simulink model "untitled"  (R2016b)
settings: Solver=VariableStepAuto  StartTime=0.0  StopTime=10.0  RelTol=1e-3
undefined symbols (not defined in the file or in its folder): h
libraries: xbsIndex_r4 x133
settings Model: Creator=rm101  LastModifiedBy=rm101

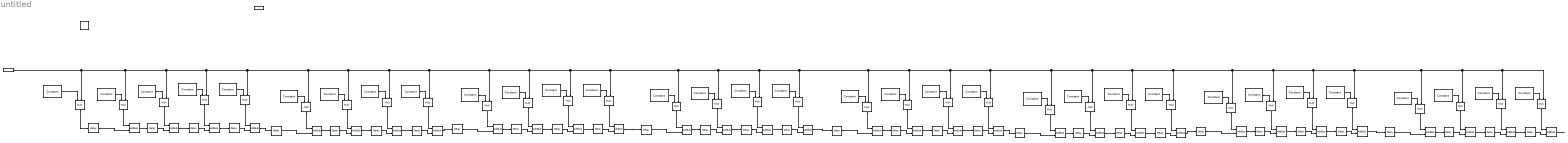
== system untitled ==
  " System Generator" : xbsIndex_r4/ System Generator  Tag=genX  xilinxfamily=Kintex7  part=xc7k325t  speed=-3  package=fbg676  synthesis_tool=Vivado  clock_wrapper=Clock Enables  directory=./netlist  proj_type=Vivado  Synth_file=Vivado Synthesis Defaults  Impl_file=Vivado Implementation Defaults  testbench=off  simulink_period=1  sysclk_period=10  dcm_input_clock_period=10  incr_netlist=off  trim_vbits=Everywhere in SubSystem  dbl_ovrd=According to Block Masks  core_generation=According to Block Masks  run_coregen=off  deprecated_control=off  eval_field=0  block_type=sysgen
  AddSub{,1..31} (32 alike) : xbsIndex_r4/AddSub  mode=Addition  use_carryin=off  use_carryout=off  en=off  latency=add1  precision=Full  arith_type=Unsigned  n_bits=16  bin_pt=14  quantization=Truncate  overflow=Wrap  use_behavioral_HDL=off  hw_selection=Fabric  pipelined=off  dbl_ovrd=off  block_type=addsub
  Constant : xbsIndex_r4/Constant  const=h(16,33)  gui_display_data_type=Fixed-point  arith_type=Signed (2's comp)  n_bits=w  bin_pt=d  preci_type=Single  exp_width=8  frac_width=24  explicit_period=off  period=1  equ=P=C  opselect=C  inp2=PCIN>>17  opr=+  inp1=P  carry=CIN  dbl_ovrd=off  block_type=constant
  Constant{1,5,9,13,17,21,28,32} (8 alike) : xbsIndex_r4/Constant  const=h(16,32)  gui_display_data_type=Fixed-point  arith_type=Signed (2's comp)  n_bits=w  bin_pt=d  preci_type=Single  exp_width=8  frac_width=24  explicit_period=off  period=1  equ=P=C  opselect=C  inp2=PCIN>>17  opr=+  inp1=P  carry=CIN  dbl_ovrd=off  block_type=constant
  Constant{2,6,10,14,18,22,25,29} (8 alike) : xbsIndex_r4/Constant  const=h(16,31)  gui_display_data_type=Fixed-point  arith_type=Signed (2's comp)  n_bits=w  bin_pt=d  preci_type=Single  exp_width=8  frac_width=24  explicit_period=off  period=1  equ=P=C  opselect=C  inp2=PCIN>>17  opr=+  inp1=P  carry=CIN  dbl_ovrd=off  block_type=constant
  Constant{3,7,11,15,19,23,26,30} (8 alike) : xbsIndex_r4/Constant  const=h(16,30)  gui_display_data_type=Fixed-point  arith_type=Signed (2's comp)  n_bits=w  bin_pt=d  preci_type=Single  exp_width=8  frac_width=24  explicit_period=off  period=1  equ=P=C  opselect=C  inp2=PCIN>>17  opr=+  inp1=P  carry=CIN  dbl_ovrd=off  block_type=constant
  Constant{4,8,12,16,20,24,27,31} (8 alike) : xbsIndex_r4/Constant  const=h(16,29)  gui_display_data_type=Fixed-point  arith_type=Signed (2's comp)  n_bits=w  bin_pt=d  preci_type=Single  exp_width=8  frac_width=24  explicit_period=off  period=1  equ=P=C  opselect=C  inp2=PCIN>>17  opr=+  inp1=P  carry=CIN  dbl_ovrd=off  block_type=constant
  Delay{,1..31} (32 alike) : xbsIndex_r4/Delay  rst=off  infoeditControl=Selection of Reset will increase slice count due to use of real FFs and instead of SRLs  en=off  latency=1  reg_retiming=off  dbl_ovrd=off  block_type=delay
  Gateway In : xbsIndex_r4/Gateway In  gui_display_data_type=Fixed-point  arith_type="Signed  (2's comp)"  n_bits=16  bin_pt=14  preci_type=Single  exp_width=8  frac_width=24  rows=1  columns=1  quantization="Round  (unbiased: +/- Inf)"  overflow=Saturate  period=1  UseAsADC=off  ADCChannel='1'  interface=None  automatic_assignment=on  address_offset=hex2dec('00')  intf_name=''  intf_description=''  default_value=0  timing_constraint=None  locs_specified=off  LOCs={}  io_standard={}  inherit_from_input=off  hdl_port=on  dbl_ovrd=off  block_type=gatewayin
  Gateway Out : xbsIndex_r4/Gateway Out  inherit_from_input=off  hdl_port=on  rows=1  columns=1  UseAsDAC=off  DACChannel='1'  interface=None  automatic_assignment=on  address_offset=hex2dec('00')  intf_name=''  intf_description=''  timing_constraint=None  locs_specified=off  LOCs={}  io_standard={}  block_type=gatewayout
  Mult{,1..32} (33 alike) : xbsIndex_r4/Mult  precision=User Defined  arith_type="Signed  (2's comp)"  n_bits=w  bin_pt=d  quantization="Round  (unbiased: +/- Inf)"  overflow=Saturate  en=off  latency=mul1  use_behavioral_HDL=off  opt=Speed  use_embedded=on  optimum_pipeline=off  pipeline=on  dbl_ovrd=off  use_rpm=on  placement_style=Triangular  block_type=mult
  wires:
  Delay/1 -> AddSub/2
  Mult/1 -> Delay/1
  Constant/1 -> Mult/1
  Mult1/1 -> AddSub/1
  Constant1/1 -> Mult1/1
  AddSub/1 -> Delay1/1
  Mult2/1 -> AddSub1/1
  Constant2/1 -> Mult2/1
  AddSub1/1 -> Delay2/1
  Mult3/1 -> AddSub2/1
  Constant3/1 -> Mult3/1
  Delay1/1 -> AddSub1/2
  Delay2/1 -> AddSub2/2
  Mult4/1 -> AddSub3/1
  Constant4/1 -> Mult4/1
  Delay3/1 -> AddSub3/2
  AddSub2/1 -> Delay3/1
  Delay4/1 -> AddSub4/2
  AddSub3/1 -> Delay4/1
  Mult5/1 -> AddSub4/1
  Constant5/1 -> Mult5/1
  AddSub4/1 -> Delay5/1
  Mult6/1 -> AddSub5/1
  Constant6/1 -> Mult6/1
  AddSub5/1 -> Delay6/1
  Mult7/1 -> AddSub6/1
  Constant7/1 -> Mult7/1
  Delay5/1 -> AddSub5/2
  Delay6/1 -> AddSub6/2
  Mult8/1 -> AddSub7/1
  Constant8/1 -> Mult8/1
  Delay7/1 -> AddSub7/2
  AddSub6/1 -> Delay7/1
  Delay8/1 -> AddSub8/2
  AddSub7/1 -> Delay8/1
  Mult9/1 -> AddSub8/1
  Constant9/1 -> Mult9/1
  AddSub8/1 -> Delay9/1
  Mult10/1 -> AddSub9/1
  Constant10/1 -> Mult10/1
  AddSub9/1 -> Delay10/1
  Mult11/1 -> AddSub10/1
  Constant11/1 -> Mult11/1
  Delay9/1 -> AddSub9/2
  Delay10/1 -> AddSub10/2
  Mult12/1 -> AddSub11/1
  Constant12/1 -> Mult12/1
  Delay11/1 -> AddSub11/2
  AddSub10/1 -> Delay11/1
  Delay12/1 -> AddSub12/2
  AddSub11/1 -> Delay12/1
  Mult13/1 -> AddSub12/1
  Constant13/1 -> Mult13/1
  AddSub12/1 -> Delay13/1
  Mult14/1 -> AddSub13/1
  Constant14/1 -> Mult14/1
  AddSub13/1 -> Delay14/1
  Mult15/1 -> AddSub14/1
  Constant15/1 -> Mult15/1
  Delay13/1 -> AddSub13/2
  Delay14/1 -> AddSub14/2
  Mult16/1 -> AddSub15/1
  Constant16/1 -> Mult16/1
  Delay15/1 -> AddSub15/2
  AddSub14/1 -> Delay15/1
  Delay16/1 -> AddSub16/2
  AddSub15/1 -> Delay16/1
  Mult17/1 -> AddSub16/1
  Constant17/1 -> Mult17/1
  AddSub16/1 -> Delay17/1
  Mult25/1 -> AddSub17/1
  Constant25/1 -> Mult25/1
  AddSub17/1 -> Delay24/1
  Mult26/1 -> AddSub24/1
  Constant26/1 -> Mult26/1
  Delay17/1 -> AddSub17/2
  Delay24/1 -> AddSub24/2
  Mult27/1 -> AddSub25/1
  Constant27/1 -> Mult27/1
  Delay25/1 -> AddSub25/2
  AddSub24/1 -> Delay25/1
  Delay26/1 -> AddSub26/2
  AddSub25/1 -> Delay26/1
  Mult28/1 -> AddSub26/1
  Constant28/1 -> Mult28/1
  AddSub26/1 -> Delay27/1
  Mult29/1 -> AddSub27/1
  Constant29/1 -> Mult29/1
  AddSub27/1 -> Delay28/1
  Mult30/1 -> AddSub28/1
  Constant30/1 -> Mult30/1
  Delay27/1 -> AddSub27/2
  Delay28/1 -> AddSub28/2
  Mult31/1 -> AddSub29/1
  Constant31/1 -> Mult31/1
  Delay29/1 -> AddSub29/2
  AddSub28/1 -> Delay29/1
  Delay30/1 -> AddSub30/2
  AddSub29/1 -> Delay30/1
  Mult32/1 -> AddSub30/1
  Constant32/1 -> Mult32/1
  AddSub30/1 -> Delay31/1
  Mult18/1 -> AddSub31/1
  Constant18/1 -> Mult18/1
  AddSub31/1 -> Delay18/1
  Mult19/1 -> AddSub18/1
  Constant19/1 -> Mult19/1
  Delay31/1 -> AddSub31/2
  Delay18/1 -> AddSub18/2
  Mult20/1 -> AddSub19/1
  Constant20/1 -> Mult20/1
  Delay19/1 -> AddSub19/2
  AddSub18/1 -> Delay19/1
  Delay20/1 -> AddSub20/2
  AddSub19/1 -> Delay20/1
  Mult21/1 -> AddSub20/1
  Constant21/1 -> Mult21/1
  AddSub20/1 -> Delay21/1
  Mult22/1 -> AddSub21/1
  Constant22/1 -> Mult22/1
  AddSub21/1 -> Delay22/1
  Mult23/1 -> AddSub22/1
  Constant23/1 -> Mult23/1
  Delay21/1 -> AddSub21/2
  Delay22/1 -> AddSub22/2
  Mult24/1 -> AddSub23/1
  Gateway In/1 -> Mult1/2, Mult5/2, Mult8/2, Mult9/2, Mult12/2, Mult13/2, Mult15/2, Mult16/2, Mult17/2, Mult28/2, Mult29/2, Mult30/2, Mult31/2, Mult32/2, Mult18/2, Mult19/2, Mult20/2, Mult21/2, Mult22/2, Mult23/2, Mult24/2, Mult27/2, Mult26/2, Mult25/2, Mult14/2, Mult11/2, Mult10/2, Mult7/2, Mult6/2, Mult4/2, Mult3/2, Mult2/2, Mult/2
  Constant24/1 -> Mult24/1
  Delay23/1 -> AddSub23/2
  AddSub23/1 -> ?
  AddSub22/1 -> Delay23/1
